simulink model "GA_LQi_sim"  (R2019a)
settings: Solver=ode4  StartTime=0.0  StopTime=param.Tsim  FixedStep=param.Ts  MaxStep=0.2  RelTol=1e-3
undefined symbols (not defined in the file or in its folder): param, sigbuilder_block
libraries: simulink x1
settings Model: Creator=yashasvi_sai  LastModifiedBy=ICS
settings SolverCC: ZeroCrossAlgorithm=Adaptive
settings DebuggingCC: IgnoredZcDiagnostic=none

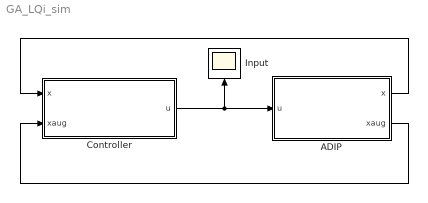
== system GA_LQi_sim ==
  ADIP : Subsystem
  Controller : Subsystem
  Input : Scope
  wires:
  ADIP/2(xaug) -> Controller/2(xaug)
  Controller/1(u) -> ADIP/1(u), Input/1
  ADIP/1(x) -> Controller/1(x)

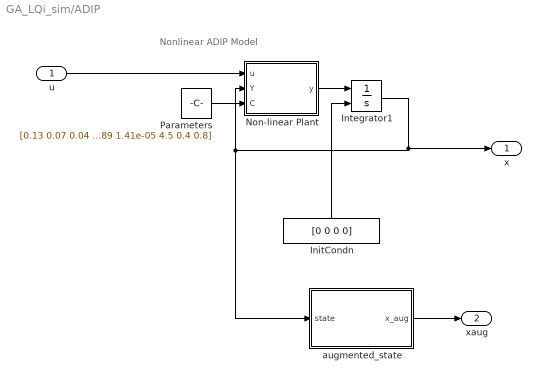
== system GA_LQi_sim/ADIP ==
  note: Nonlinear ADIP Model
  u : Inport
  InitCondn : Constant  Value=[0 0 0 0]
  Integrator1 : Integrator  InitialConditionSource=external  InitialCondition=param.theta0
  "Non-linear Plant " : MATLAB Function  TreatAsAtomicUnit=on
  Parameters : Constant  Value=[0.13 0.07 0.04 0.154 0.186 -9.81 0.0003 0.000202 0.00015814 0.000737 0.00289 1.41e-05 4.5 0.4 0.8]
  augmented_state : Subsystem
  x : Outport
  xaug : Outport  Port=2
  wires:
  "Non-linear Plant "/1(y) -> Integrator1/1
  Integrator1/1 -> augmented_state/1(state), "Non-linear Plant "/2(Y), x/1
  u/1 -> "Non-linear Plant "/1(u)
  Parameters/1 -> "Non-linear Plant "/3(C)
  augmented_state/1(x_aug) -> xaug/1
  InitCondn/1 -> Integrator1/2

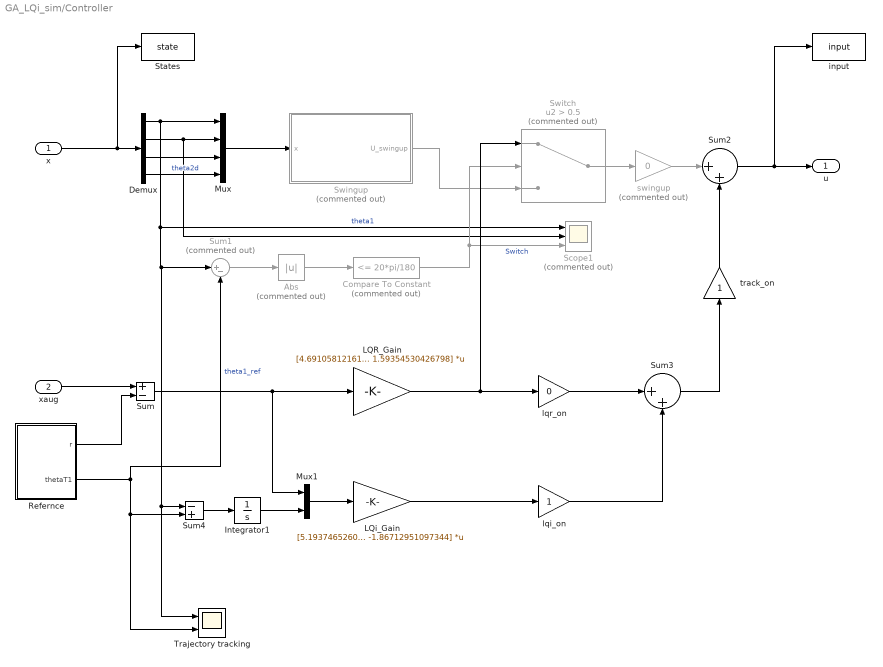
== system GA_LQi_sim/Controller ==
  x : Inport
  xaug : Inport  Port=2
  Abs : Abs  Commented=on
  Compare To Constant : simulink/Logic and Bit Operations/Compare To Constant  Commented=on  relop=<=  const=20*pi/180  OutDataTypeStr=boolean
  Demux : Demux
  Integrator1 : Integrator
  LQR_Gain : Gain  Gain=[4.69105812161154 14.9392898979114 1.33286732839246 1.59354530426798]  Multiplication=Matrix(K*u)
  LQi_Gain : Gain  Gain=[5.1937465260465 15.5114677034942 1.39662706176635 1.65359146034935 -1.86712951097344]  Multiplication=Matrix(K*u)
  Mux : Mux
  Mux1 : Mux  Inputs=2
  Refernce : Subsystem
  Scope1 : Scope  Commented=on  NumInputPorts=3
  States : ToWorkspace  VariableName=state  SampleTime=-1
  Sum : Sum  Inputs=+-
  Sum1 : Sum  Commented=on  Inputs=|+-
  Sum2 : Sum  Inputs=|++
  Sum3 : Sum  Inputs=|++
  Sum4 : Sum  Inputs=-+
  Swingup : Subsystem  Commented=on
  Switch : Switch  Commented=on  Criteria=u2 > Threshold  Threshold=0.5
  Trajectory tracking : Scope  NumInputPorts=2
  input : ToWorkspace  VariableName=input  SampleTime=-1
  lqi_on : Gain
  lqr_on : Gain  Gain=0
  swingup : Gain  Commented=on  Gain=0
  track_on : Gain
  u : Outport
  wires:
  x/1 -> States/1, Demux/1
  Demux/1 -> Scope1/1, Trajectory tracking/1, Sum4/1, Sum1/1, Mux/1  "theta1"
  Swingup/1(U_swingup) -> Switch/3
  Sum/1 -> Mux1/1, LQR_Gain/1
  Refernce/1(r) -> Sum/2
  Abs/1 -> Compare To Constant/1
  Demux/3 -> Mux/3
  Demux/2 -> Scope1/2, Mux/2
  Demux/4 -> Mux/4  "theta2d"
  Mux/1 -> Swingup/1(x)
  Sum1/1 -> Abs/1
  Compare To Constant/1 -> Scope1/3, Switch/2  "Switch"
  xaug/1 -> Sum/1
  Refernce/2(thetaT1) -> Sum1/2, Trajectory tracking/2, Sum4/2  "theta1_ref"
  Sum4/1 -> Integrator1/1
  Mux1/1 -> LQi_Gain/1
  Integrator1/1 -> Mux1/2
  lqi_on/1 -> Sum3/2
  LQi_Gain/1 -> lqi_on/1
  Sum3/1 -> track_on/1
  Sum2/1 -> input/1, u/1
  lqr_on/1 -> Sum3/1
  LQR_Gain/1 -> lqr_on/1, Switch/1
  Switch/1 -> swingup/1
  swingup/1 -> Sum2/1
  track_on/1 -> Sum2/2

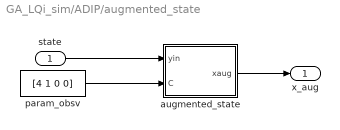
== system GA_LQi_sim/ADIP/augmented_state ==
  state : Inport
  augmented_state : MATLAB Function  TreatAsAtomicUnit=on
  param_obsv : Constant  Value=[4 1 0 0]
  x_aug : Outport
  wires:
  param_obsv/1 -> augmented_state/2(C)
  state/1 -> augmented_state/1(yin)
  augmented_state/1(xaug) -> x_aug/1

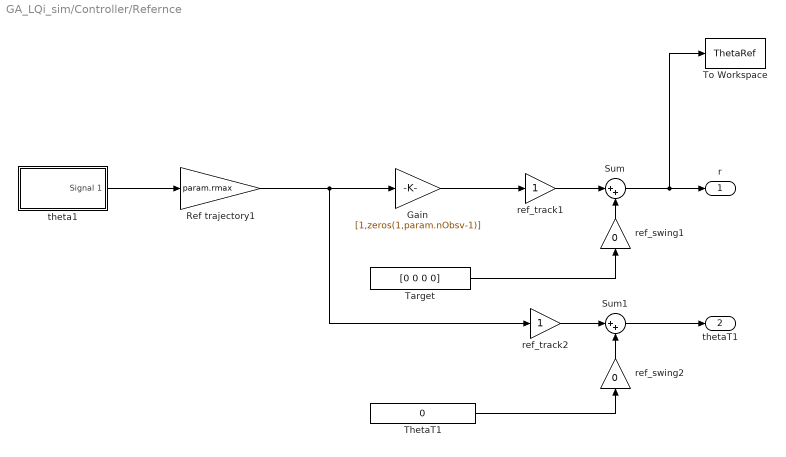
== system GA_LQi_sim/Controller/Refernce ==
  Gain : Gain  Gain=[1,zeros(1,param.nObsv-1)]
  Ref trajectory1 : Gain  Gain=param.rmax
  Sum : Sum  Inputs=|++
  Sum1 : Sum  Inputs=|++
  Target : Constant  Value=[0 0 0 0]
  ThetaT1 : Constant  Value=0
  To Workspace : ToWorkspace  VariableName=ThetaRef  SampleTime=-1
  ref_swing1 : Gain  Gain=0
  ref_swing2 : Gain  Gain=0
  ref_track1 : Gain
  ref_track2 : Gain
  theta1 : Subsystem  Tag=STV Subsys  LoadFcn=sigbuilder_block('load');  StartFcn=sigbuilder_block('start');  StopFcn=sigbuilder_block('stop');  ClipboardFcn=sigbuilder_block('clipboard');  mask(Sigbuilder block){tuvar=[0:10]}
      mask help: Simulink:masks:SigbuilderBlock_MD
      mask init:
      | if ~strcmp(get_param(bdroot(gcbh),'SimulationStatus'),'stopped') tuvar = sigbuilder_block('maskInit'); end
      settings: CopyFcn=sigbuilder_block('copy');  DeleteFcn=sigbuilder_block('delete');  ModelCloseFcn=sigbuilder_block('modelClose');  PreSaveFcn=sigbuilder_block('preSave');  PauseFcn=sigbuilder_block('pause');  ContinueFcn=sigbuilder_block('continue');  NameChangeFcn=sigbuilder_block('namechange');  OpenFcn=sigbuilder_block('open',[5.5 30 1909 958 ]);  CloseFcn=sigbuilder_block('close');
      mask Display: plot(0, 0, 100, 100,[2, 2, 32, 32, 2], [68, 8, 8, 68, 68],[32, 2], [38, 38], [32, 19, 2],[53, 60, 44], [32, 17, 17, 2],[16, 16, 31, 31]);txt = getActiveGroup(gcbh);text(2, 100, txt,'verticalAlignment', 'top');
  r : Outport
  thetaT1 : Outport  Port=2
  wires:
  Sum/1 -> To Workspace/1, r/1
  ref_track2/1 -> Sum1/1
  ThetaT1/1 -> ref_swing2/1
  ref_swing1/1 -> Sum/2
  Gain/1 -> ref_track1/1
  Ref trajectory1/1 -> Gain/1, ref_track2/1
  ref_track1/1 -> Sum/1
  Target/1 -> ref_swing1/1
  Sum1/1 -> thetaT1/1
  ref_swing2/1 -> Sum1/2
  theta1/1(Signal 1) -> Ref trajectory1/1

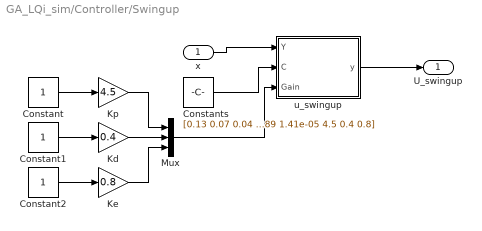
== system GA_LQi_sim/Controller/Swingup ==
  x : Inport
  Constant : Constant
  Constant1 : Constant
  Constant2 : Constant
  Constants : Constant  Value=[0.13 0.07 0.04 0.154 0.186 -9.81 0.0003 0.000202 0.00015814 0.000737 0.00289 1.41e-05 4.5 0.4 0.8]
  Kd : Gain  Gain=0.4
  Ke : Gain  Gain=0.8
  Kp : Gain  Gain=4.5
  Mux : Mux  Inputs=3
  "u_swingup " : MATLAB Function  TreatAsAtomicUnit=on
  U_swingup : Outport
  wires:
  x/1 -> "u_swingup "/1(Y)
  Constants/1 -> "u_swingup "/2(C)
  "u_swingup "/1(y) -> U_swingup/1
  Constant/1 -> Kp/1
  Constant1/1 -> Kd/1
  Constant2/1 -> Ke/1
  Kp/1 -> Mux/1
  Kd/1 -> Mux/2
  Ke/1 -> Mux/3
  Mux/1 -> "u_swingup "/3(Gain)

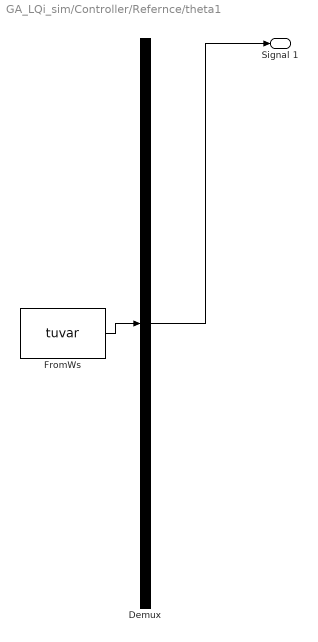
== system GA_LQi_sim/Controller/Refernce/theta1 ==
  Demux : Demux  Tag=STV Demux  Outputs=1
  FromWs : FromWorkspace  Tag=STV FromWs  VariableName=tuvar  SampleTime=0
      SigBuilderData=|
      | common.afterFinalStr = 'Extrapolate'
      | common.sampleTime = 0
      | dataSet.timeRange = [0 50]
      | dataSet.name = 'Group 1'
      | sbobj.Groups.Name = 'Group 1'
      | sbobj.Groups.Signals.Name = 'Signal 1'
      | sbobj.Groups.Signals.XData = [0 2 5 6.5 10.5 12 15 50]
      | sbobj.Groups.Signals.YData = [0 0.005 1 1 -1.005 -1 0 0]
      | sbobj.Groups.TimeRange = [0 50]
  Signal 1 : Outport  Tag=STV Outport
  wires:
  Demux/1 -> Signal 1/1
  FromWs/1 -> Demux/1

== matlab function GA_LQi_sim/Controller/Swingup/u_swingup  ==
  data: Y input; y output; C input; Gain input
function y = fcn(Y, C, Gain)
m1=C(1); % Mass of arm
m2=C(2); % Mass of pendulum
mh = C(3); % Mass of Hinge
l1  = C(4); % Length of arm
l2 = C(5); % Length of pendulum
g_ = C(6);
J_arm = C(7);
J_pend = C(8);
J_motor = C(9);
J_sensor = C(10);
fv1 = C(11);
fv2 = C(12);

y1 = Y(1);  % actual theta1          
y2 = Y(2);  % actual theta2
y3 = Y(3);  % actual theta1d
y4 = Y(4);  % actual theta2d

Kp = Gain(1);
Kd = Gain(2);
Ke = Gain(3);

y1_tilda = Y(1);

u_swing = (Kd*(J_pend*fv1*y3 + (fv1*l2^2*m2*y3)/4 + (l1^2*l2^2*m2^2*y3^2*sin(2*y1 - 2*y2))/8 + (l1*l2^3*m2^2*y4^2*sin(y1 - y2))/8 + (g_*l1*l2^2*m2^2*sin(y1))/8 + (J_pend*g_*l1*m1*sin(y1))/2 + J_pend*g_*l1*m2*sin(y1) + J_pend*g_*l1*mh*sin(y1) + (g_*l1*l2^2*m2^2*sin(y1 - 2*y2))/8 - (fv2*l1*l2*m2*y4*cos(y1 - y2))/2 + (g_*l1*l2^2*m1*m2*sin(y1))/8 + (g_*l1*l2^2*m2*mh*sin(y1))/4 + (J_pend*l1*l2*m2*y4^2*sin(y1 - y2))/2) - (y3 + Kp*y1_tilda)*(J_arm*J_pend + J_motor*J_pend + J_pend*J_sensor + (l1^2*l2^2*m2^2)/4 + (J_arm*l2^2*m2)/4 + (J_motor*l2^2*m2)/4 + (J_pend*l1^2*m1)/4 + J_pend*l1^2*m2 + (J_sensor*l2^2*m2)/4 - (l1^2*l2^2*m2^2*cos(y1 - y2)^2)/4 + (l1^2*l2^2*m1*m2)/16))/(Kd*((m2*l2^2)/4 + J_pend) + Ke*((J_arm*y3^2)/2 + (J_motor*y3^2)/2 + (J_pend*y4^2)/2 + (J_sensor*y3^2)/2 + g_*m1*(l1/2 - (l1*cos(y1))/2) + g_*m2*(l1 + l2/2 - l1*cos(y1) - (l2*cos(y2))/2) + g_*mh*(l1 - l1*cos(y1)))*(J_arm*J_pend + J_motor*J_pend + J_pend*J_sensor + (l1^2*l2^2*m2^2)/4 + (J_arm*l2^2*m2)/4 + (J_motor*l2^2*m2)/4 + (J_pend*l1^2*m1)/4 + J_pend*l1^2*m2 + (J_sensor*l2^2*m2)/4 - (l1^2*l2^2*m2^2*cos(y1 - y2)^2)/4 + (l1^2*l2^2*m1*m2)/16));
y = u_swing;

== matlab function GA_LQi_sim/ADIP/Non-linear Plant  ==
  data: u input; Y input; y output; C input
function y = fcn(u,Y,C)
m1=C(1); % Mass of arm
m2=C(2); % Mass of pendulum
mh = C(3); % Mass of Hinge
l1  = C(4); % Length of arm
l2 = C(5); % Length of pendulum
g_ = C(6);
J_arm = C(7);
J_pend = C(8);
J_motor = C(9);
J_sensor = C(10);
fv1 = C(11);
fv2 = C(12);

y1 = Y(1);  % actual theta1          
y2 = Y(2);  % actual theta2
y3 = Y(3);  % actual theta1d
y4 = Y(4);  % actual theta2d

dy1 = y3;
dy2 = y4;
dy3 =-(2*(8*J_pend*fv1*y3 - 2*l2^2*m2*u - 8*J_pend*u + 2*fv1*l2^2*m2*y3 + l1^2*l2^2*m2^2*y3^2*sin(2*y1 - 2*y2) + l1*l2^3*m2^2*y4^2*sin(y1 - y2) + g_*l1*l2^2*m2^2*sin(y1) + 4*J_pend*g_*l1*m1*sin(y1) + 8*J_pend*g_*l1*m2*sin(y1) + 8*J_pend*g_*l1*mh*sin(y1) + g_*l1*l2^2*m2^2*sin(y1 - 2*y2) - 4*fv2*l1*l2*m2*y4*cos(y1 - y2) + g_*l1*l2^2*m1*m2*sin(y1) + 2*g_*l1*l2^2*m2*mh*sin(y1) + 4*J_pend*l1*l2*m2*y4^2*sin(y1 - y2)))/(16*J_arm*J_pend + 16*J_motor*J_pend + 16*J_pend*J_sensor + 4*l1^2*l2^2*m2^2 + 4*J_arm*l2^2*m2 + 4*J_motor*l2^2*m2 + 4*J_pend*l1^2*m1 + 16*J_pend*l1^2*m2 + 4*J_sensor*l2^2*m2 - 4*l1^2*l2^2*m2^2*cos(y1 - y2)^2 + l1^2*l2^2*m1*m2);
dy4 =(2*(l1^2*l2^2*m2^2*y4^2*sin(2*y1 - 2*y2) - 8*J_motor*fv2*y4 - 8*J_sensor*fv2*y4 - 2*fv2*l1^2*m1*y4 - 8*fv2*l1^2*m2*y4 - 8*J_arm*fv2*y4 - 4*l1*l2*m2*u*cos(y1 - y2) + 2*g_*l1^2*l2*m2^2*sin(2*y1 - y2) + 4*l1^3*l2*m2^2*y3^2*sin(y1 - y2) - 2*g_*l1^2*l2*m2^2*sin(y2) - 4*J_arm*g_*l2*m2*sin(y2) - 4*J_motor*g_*l2*m2*sin(y2) - 4*J_sensor*g_*l2*m2*sin(y2) + g_*l1^2*l2*m1*m2*sin(2*y1 - y2) + 2*g_*l1^2*l2*m2*mh*sin(2*y1 - y2) + l1^3*l2*m1*m2*y3^2*sin(y1 - y2) + 4*fv1*l1*l2*m2*y3*cos(y1 - y2) + 2*g_*l1^2*l2*m2*mh*sin(y2) + 4*J_arm*l1*l2*m2*y3^2*sin(y1 - y2) + 4*J_motor*l1*l2*m2*y3^2*sin(y1 - y2) + 4*J_sensor*l1*l2*m2*y3^2*sin(y1 - y2)))/(16*J_arm*J_pend + 16*J_motor*J_pend + 16*J_pend*J_sensor + 2*l1^2*l2^2*m2^2 + 4*J_arm*l2^2*m2 + 4*J_motor*l2^2*m2 + 4*J_pend*l1^2*m1 + 16*J_pend*l1^2*m2 + 4*J_sensor*l2^2*m2 - 2*l1^2*l2^2*m2^2*cos(2*y1 - 2*y2) + l1^2*l2^2*m1*m2);
y = [dy1 dy2 dy3 dy4]';

== matlab function GA_LQi_sim/ADIP/augmented_state/augmented_state ==
  data: yin input; xaug output; C input
function xaug = fcn(yin,C)

% x1 = yin(1); x2 = yin(2); x3 = yin(3); x4 = yin(4);
% 
% 
% % P = size(param.A,1);
% 
% % switch P
% %     case 4
% %         Psi = []; % 4 just the states
% %     case 6 
% %         Psi = [sin(x1).*cos(x1) ones(size(x1,1),1)];  % 6 - sin*cos
% %     case 7
% %         Psi = [sin(x1) cos(x1) ones(size(x1,1),1)];  % 7 - states + sin and cos
% %     case 8
% %         Psi = [sin(x1) cos(x1) sin(x1).*cos(x1) ones(size(x1,1),1)];  % 8 - states + sin,cos and sin*cos
% %     case 12 
% %         Psi = [x1.^2 x3.^2 x1.*x2 x1.*x3 x1.*x4 x2.*x3 x3.*x4 ones(size(x1,1),1)];  % 12 - only Poly without x2^2 and x4^2
% %     case 19
% %           Psi = [x1.^2 x3.^2 x1.*x2 x1.*x3 x1.*x4 x2.*x3 x3.*x4...
% %     x1.*sin(x1) x3.*sin(x2) x1.^2.*sin(x1) x3.^2.*sin(x2) sin(x1) cos(x1)...
% %     sin(x1).*cos(x1) ones(size(x1,1),1)];  % 19
% % end
% 
% % Psi = [ x1.^2, x1.*x2, x1.*x3, x1.*x4, x2.^2, x2.*x3, x2.*x4, x4.^2, sin(x1), sin(x2), cos(x1), cos(x2), cos(x1).*sin(x1), cos(x2).*sin(x1), cos(x1).*sin(x2), cos(x2).*sin(x2), x1.^2.*sin(x1), x1.^2.*sin(x2), x1.^2.*cos(x1), x1.^2.*cos(x2), x1.*x2.*sin(x1), x1.*x2.*cos(x1), x1.*x2.*cos(x2), x1.*x3.*sin(x1), x1.*x3.*sin(x2), x1.*x3.*cos(x1), x1.*x3.*cos(x2), x1.*x4.*sin(x1), x1.*x4.*sin(x2), x1.*x4.*cos(x1), x1.*x4.*cos(x2), x2.^2.*sin(x1), x2.^2.*sin(x2), x2.^2.*cos(x1), x2.^2.*cos(x2), x2.*x3.*sin(x1), x2.*x3.*sin(x2), x2.*x3.*cos(x1), x2.*x3.*cos(x2), x2.*x4.*sin(x1), x2.*x4.*sin(x2), x2.*x4.*cos(x1), x2.*x4.*cos(x2), x3.*x4.*sin(x2), x3.*x4.*cos(x1)];
% % Psi = [ x2.^2.*sin(2.*x1), x2.^2.*sin(2.*x2), x2.^2.*cos(2.*x1), x2.^2.*cos(2.*x2), x1.^2.*sin(2.*x1).^2, x1.^2.*cos(2.*x1).^2, x1.^2.*cos(2.*x2).^2, x1.*x2.*sin(2.*x1).^2, x1.*x2.*cos(2.*x1).^2, x1.*x2.*cos(2.*x2).^2, x2.^2.*sin(2.*x1).^2, x2.^2.*sin(2.*x2).^2, x2.^2.*cos(2.*x2).^2];
% Psi = [x1, x2, x3, x4, x1.^2.*sin(x1), x1.^2.*sin(x2), x1.^2.*cos(x1), x1.^2.*cos(x2), x1.^2.*sin(2.*x1), x1.^2.*sin(2.*x2), x1.^2.*cos(2.*x1), x1.^2.*cos(2.*x2), x1.*x2.*sin(x1), x1.*x2.*sin(x2), x1.*x2.*cos(x1), x1.*x2.*cos(x2), x1.*x2.*sin(2.*x1), x1.*x2.*sin(2.*x2), x1.*x2.*cos(2.*x1), x1.*x2.*cos(2.*x2), x2.^2.*sin(x1), x2.^2.*sin(x2), x2.^2.*cos(x1), x2.^2.*cos(x2), x2.^2.*sin(2.*x1), x2.^2.*sin(2.*x2), x2.^2.*cos(2.*x1), x2.^2.*cos(2.*x2), x1.^2.*sin(2.*x1).^2, x1.^2.*sin(2.*x2).^2, x1.^2.*cos(2.*x2).^2, x1.*x2.*sin(2.*x2).^2, x1.*x2.*cos(2.*x1).^2, x1.*x2.*cos(2.*x2).^2, x2.^2.*sin(2.*x1).^2, x2.^2.*sin(2.*x2).^2, x2.^2.*cos(2.*x1).^2];
% 
% xaug = Psi';
% switch C
%     case 1
%         Psi = []; % 4 just the states
%     case 2 
%         Psi = [sin(x1).*cos(x1) ones(size(x1,1),1)];  % 6 - sin*cos
% %     case 3
%         Psi = [sin(x1) cos(x1) ones(size(x1,1),1)];  % 7 - states + sin and cos
% %     case 4
%         Psi = [sin(x1) cos(x1) sin(x1).*cos(x1) ones(size(x1,1),1)];  % 8 - states + sin,cos and sin*cos
%     case 5 
%         Psi = [x1.^2 x3.^2 x1.*x2 x1.*x3 x1.*x4 x2.*x3 x3.*x4 ones(size(x1,1),1)];  % 12 - only Poly without x2^2 and x4^2
%     case 6
%           Psi = [x1.^2 x3.^2 x1.*x2 x1.*x3 x1.*x4 x2.*x3 x3.*x4...
%     x1.*sin(x1) x3.*sin(x2) x1.^2.*sin(x1) x3.^2.*sin(x2) sin(x1) cos(x1)...
%     sin(x1).*cos(x1) ones(size(x1,1),1)];  % 19
% Psi = [x1.^2 x3.^2 x1.*x2 x1.*x3 x1.*x4 x2.*x3 x3.*x4 ones(size(x1,1),1)];  % 12 - only Poly without x2^2 and x4^2
% 
% % end
% 
% xaug = [x1 x2 x3 x4 Psi]';

yin = yin'; nVars = C(1); polyorder = C(2); usesine = C(3); polysine = C(4);
% nObsv = C(5);

y = zeros(1,4);
ind = 1;

% poly order 1
for i=1:nVars
    y(:,ind) = yin(:,i);
    ind = ind+1;
end

if(polyorder>=2)
    % poly order 2
    for i=1:nVars
        for j=i:nVars
            y(:,ind) = yin(:,i).*yin(:,j);
            ind = ind+1;
        end
    end
end

xaug = y';

% 
% % n = size(yin,1);
% % yout = zeros(1,4);
% % ind = 1;
% % % poly order 0
% % % yout(:,ind) = ones(n,1);
% % % ind = ind+1;
% % 
% 
% % 
% 
% % 
% % if(polyorder>=3)
% %     % poly order 3
% %     for i=1:nVars
% %         for j=i:nVars
% %             for k=j:nVars
% %                 yout(:,ind) = yin(:,i).*yin(:,j).*yin(:,k);
% %                 ind = ind+1;
% %             end
% %         end
% %     end
% % end
% % 
% % if(polyorder>=4)
% %     % poly order 4
% %     for i=1:nVars
% %         for j=i:nVars
% %             for k=j:nVars
% %                 for l=k:nVars
% %                     yout(:,ind) = yin(:,i).*yin(:,j).*yin(:,k).*yin(:,l);
% %                     ind = ind+1;
% %                 end
% %             end
% %         end
% %     end
% % end
% % 
% % if(polyorder>=5)
% %     % poly order 5
% %     for i=1:nVars
% %         for j=i:nVars
% %             for k=j:nVars
% %                 for l=k:nVars
% %                     for m=l:nVars
% %                         yout(:,ind) = yin(:,i).*yin(:,j).*yin(:,k).*yin(:,l).*yin(:,m);
% %                         ind = ind+1;
% %                     end
% %                 end
% %             end
% %         end
% %     end
% % end
% % 
% % % if(usesine)
% % %     for k=1:10
% % %         yout = [yout sin(k*yin) cos(k*yin)];
% % %     end
% % % end
% % % 
% % % if(polysine)
% % %     for i=1:nVars
% % %         for k= 1:10
% % %             yout = [yout yin(:,i).*sin(k*yin) yin(:,i).*cos(k*yin)];
% % %         end
% % %     end
% % % end
% % 
% % if(usesine)
% %     for k=1:2
% %         yout = [yout sin(k*yin(:,1:2)) cos(k*yin(:,1:2))];
% %     end
% % end
% % 
% % if(polysine)
% %     for i=1:nVars
% %         for k= 1:2
% %             yout = [yout yin(:,i).*sin(k*yin(:,1:2)) yin(:,i).*cos(k*yin(:,1:2))];
% %         end
% %     end
% % end
% % 
% % if(polysine)
% %     for i=1:nVars
% %         for j= 1:nVars
% %             for k= 1:2
% %                 yout = [yout yin(:,i).*yin(:,j).*sin(k*yin(:,1:2)) yin(:,i).*yin(:,j).*cos(k*yin(:,1:2))];
% %             end
% %         end
% %     end
% % end
% % 
% % y = yout';
